simulink model "WorkingModel"  (R2023b)
settings: Solver=FixedStepDiscrete  StartTime=0.0  StopTime=param_sim_time  FixedStep=1/fs  MaxStep=1/fs  RelTol=1e-3
undefined symbols (not defined in the file): analyses, fdesignblkfcn, fs, gcbh, param_tot_samples
libraries: dspstat3 x13, SCGAnalysis_SignalGenerationLib x2
(part 2 of 20)

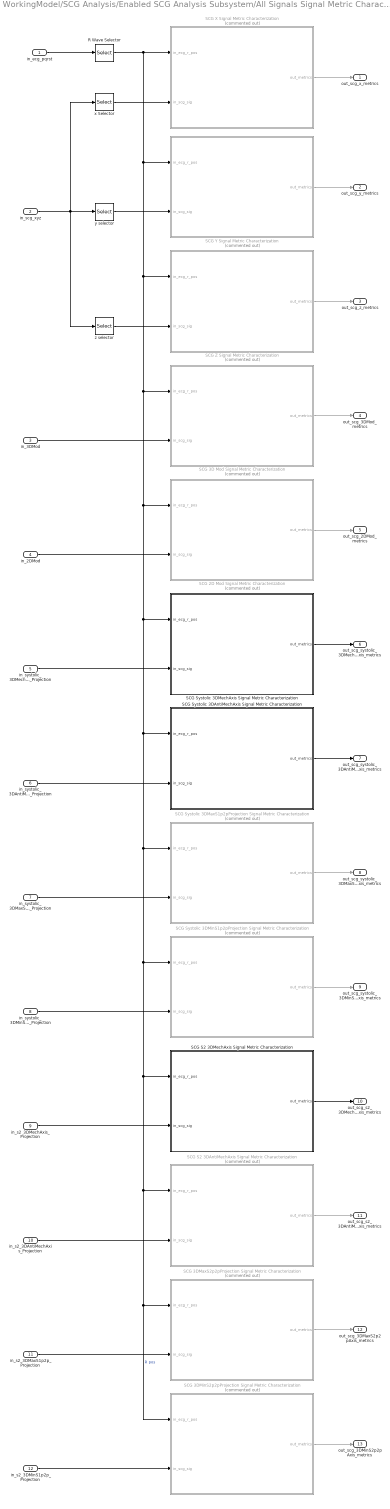
== system WorkingModel/SCG Analysis/Enabled SCG Analysis Subsystem/All Signals Signal Metric Characterization ==
  in_ecg_pqrst : Inport
  in_scg_xyz : Inport  Port=2
  in_3DMod : Inport  Port=3
  in_2DMod : Inport  Port=4
  in_systolic_3DMechAxis_Projection : Inport  Port=5
  in_systolic_3DAntiMechAxis_Projection : Inport  Port=6
  in_systolic_3DMaxS1p2p_Projection : Inport  Port=7
  in_systolic_3DMinS1p2p_Projection : Inport  Port=8
  in_s2_3DMechAxis_Projection : Inport  Port=9
  in_s2_3DAntiMechAxis_Projection : Inport  Port=10
  in_s2_3DMaxS1p2p_Projection : Inport  Port=11
  in_s2_3DMinS1p2p_Projection : Inport  Port=12
  R Wave Selector : Selector  NumberOfDimensions=2  InputPortWidth=3  IndexOptions=Select all,Index vector (dialog)  Indices=[1 3],3  OutputSizes=1,1
  SCG 2D Mod Signal Metric Characterization : Subsystem  Commented=on  mask{s1p2p_flag=on, s2p2p_flag=on, snr_flag=on, var_flag=on, morphvar_flag=on, nsd_flag=off}
      mask prompts: s1p2p_flag "S1 peak-to-peak Amplitude"; s2p2p_flag "S2 peak-to-peak Amplitude"; snr_flag "Signal-to-nose Ratio (can be further specified inside block)"; var_flag "Variance"; morphvar_flag "Cycle-to-cycle Morphological Variability"; nsd_flag "Normalized Spectral Distribution (can be further specified inside block)"
      mask DialogControl DescGroupVar Prompt: Signal Characterization
      mask DialogControl DescTextVar Prompt: SCG Signal Characterization block. Select which signal characterization metrics to evaluate:
      mask Display: image('C:\Users\Rafael\Dropbox\Post-Doc Research\Characterization.png'); % Use "Edit Image" on toolstrip to change.
  SCG 3D Mod Signal Metric Characterization : Subsystem  Commented=on  mask{s1p2p_flag=on, s2p2p_flag=on, snr_flag=on, var_flag=on, morphvar_flag=on, nsd_flag=off}
      mask prompts: s1p2p_flag "S1 peak-to-peak Amplitude"; s2p2p_flag "S2 peak-to-peak Amplitude"; snr_flag "Signal-to-nose Ratio (can be further specified inside block)"; var_flag "Variance"; morphvar_flag "Cycle-to-cycle Morphological Variability"; nsd_flag "Normalized Spectral Distribution (can be further specified inside block)"
      mask DialogControl DescGroupVar Prompt: Signal Characterization
      mask DialogControl DescTextVar Prompt: SCG Signal Characterization block. Select which signal characterization metrics to evaluate:
      mask Display: image('C:\Users\Rafael\Dropbox\Post-Doc Research\Characterization.png'); % Use "Edit Image" on toolstrip to change.
  SCG 3DMaxS2p2pProjection Signal Metric Characterization : Subsystem  Commented=on  mask{s1p2p_flag=on, s2p2p_flag=on, snr_flag=on, var_flag=on, morphvar_flag=on, nsd_flag=on}
      mask prompts: s1p2p_flag "S1 peak-to-peak Amplitude"; s2p2p_flag "S2 peak-to-peak Amplitude"; snr_flag "Signal-to-nose Ratio (can be further specified inside block)"; var_flag "Variance"; morphvar_flag "Cycle-to-cycle Morphological Variability"; nsd_flag "Normalized Spectral Distribution (can be further specified inside block)"
      mask DialogControl DescGroupVar Prompt: Signal Characterization
      mask DialogControl DescTextVar Prompt: SCG Signal Characterization block. Select which signal characterization metrics to evaluate:
      mask Display: image('C:\Users\Rafael\Dropbox\Post-Doc Research\Characterization.png'); % Use "Edit Image" on toolstrip to change.
  SCG 3DMinS2p2pProjection Signal Metric Characterization : Subsystem  Commented=on  mask{s1p2p_flag=on, s2p2p_flag=on, snr_flag=on, var_flag=on, morphvar_flag=on, nsd_flag=on}
      mask prompts: s1p2p_flag "S1 peak-to-peak Amplitude"; s2p2p_flag "S2 peak-to-peak Amplitude"; snr_flag "Signal-to-nose Ratio (can be further specified inside block)"; var_flag "Variance"; morphvar_flag "Cycle-to-cycle Morphological Variability"; nsd_flag "Normalized Spectral Distribution (can be further specified inside block)"
      mask DialogControl DescGroupVar Prompt: Signal Characterization
      mask DialogControl DescTextVar Prompt: SCG Signal Characterization block. Select which signal characterization metrics to evaluate:
      mask Display: image('C:\Users\Rafael\Dropbox\Post-Doc Research\Characterization.png'); % Use "Edit Image" on toolstrip to change.
  SCG S2 3DAntiMechAxis Signal Metric Characterization : Subsystem  Commented=on  mask{s1p2p_flag=on, s2p2p_flag=on, snr_flag=on, var_flag=on, morphvar_flag=on, nsd_flag=on}
      mask prompts: s1p2p_flag "S1 peak-to-peak Amplitude"; s2p2p_flag "S2 peak-to-peak Amplitude"; snr_flag "Signal-to-nose Ratio (can be further specified inside block)"; var_flag "Variance"; morphvar_flag "Cycle-to-cycle Morphological Variability"; nsd_flag "Normalized Spectral Distribution (can be further specified inside block)"
      mask DialogControl DescGroupVar Prompt: Signal Characterization
      mask DialogControl DescTextVar Prompt: SCG Signal Characterization block. Select which signal characterization metrics to evaluate:
      mask Display: image('C:\Users\Rafael\Dropbox\Post-Doc Research\Characterization.png'); % Use "Edit Image" on toolstrip to change.
  SCG S2 3DMechAxis Signal Metric Characterization : Subsystem  mask{s1p2p_flag=on, s2p2p_flag=on, snr_flag=on, var_flag=on, morphvar_flag=on, nsd_flag=on}
      mask prompts: s1p2p_flag "S1 peak-to-peak Amplitude"; s2p2p_flag "S2 peak-to-peak Amplitude"; snr_flag "Signal-to-nose Ratio (can be further specified inside block)"; var_flag "Variance"; morphvar_flag "Cycle-to-cycle Morphological Variability"; nsd_flag "Normalized Spectral Distribution (can be further specified inside block)"
      mask DialogControl DescGroupVar Prompt: Signal Characterization
      mask DialogControl DescTextVar Prompt: SCG Signal Characterization block. Select which signal characterization metrics to evaluate:
      mask Display: image('C:\Users\Rafael\Dropbox\Post-Doc Research\Characterization.png'); % Use "Edit Image" on toolstrip to change.
  SCG Systolic 3DAntiMechAxis Signal Metric Characterization : Subsystem  mask{s1p2p_flag=on, s2p2p_flag=on, snr_flag=on, var_flag=on, morphvar_flag=on, nsd_flag=on}
      mask prompts: s1p2p_flag "S1 peak-to-peak Amplitude"; s2p2p_flag "S2 peak-to-peak Amplitude"; snr_flag "Signal-to-nose Ratio (can be further specified inside block)"; var_flag "Variance"; morphvar_flag "Cycle-to-cycle Morphological Variability"; nsd_flag "Normalized Spectral Distribution (can be further specified inside block)"
      mask DialogControl DescGroupVar Prompt: Signal Characterization
      mask DialogControl DescTextVar Prompt: SCG Signal Characterization block. Select which signal characterization metrics to evaluate:
      mask Display: image('C:\Users\Rafael\Dropbox\Post-Doc Research\Characterization.png'); % Use "Edit Image" on toolstrip to change.
  SCG Systolic 3DMaxS1p2pProjection Signal Metric Characterization : Subsystem  Commented=on  mask{s1p2p_flag=on, s2p2p_flag=on, snr_flag=on, var_flag=on, morphvar_flag=on, nsd_flag=on}
      mask prompts: s1p2p_flag "S1 peak-to-peak Amplitude"; s2p2p_flag "S2 peak-to-peak Amplitude"; snr_flag "Signal-to-nose Ratio (can be further specified inside block)"; var_flag "Variance"; morphvar_flag "Cycle-to-cycle Morphological Variability"; nsd_flag "Normalized Spectral Distribution (can be further specified inside block)"
      mask DialogControl DescGroupVar Prompt: Signal Characterization
      mask DialogControl DescTextVar Prompt: SCG Signal Characterization block. Select which signal characterization metrics to evaluate:
      mask Display: image('C:\Users\Rafael\Dropbox\Post-Doc Research\Characterization.png'); % Use "Edit Image" on toolstrip to change.
  SCG Systolic 3DMechAxis Signal Metric Characterization : Subsystem  mask{s1p2p_flag=on, s2p2p_flag=on, snr_flag=on, var_flag=on, morphvar_flag=on, nsd_flag=on}
      mask prompts: s1p2p_flag "S1 peak-to-peak Amplitude"; s2p2p_flag "S2 peak-to-peak Amplitude"; snr_flag "Signal-to-nose Ratio (can be further specified inside block)"; var_flag "Variance"; morphvar_flag "Cycle-to-cycle Morphological Variability"; nsd_flag "Normalized Spectral Distribution (can be further specified inside block)"
      mask DialogControl DescGroupVar Prompt: Signal Characterization
      mask DialogControl DescTextVar Prompt: SCG Signal Characterization block. Select which signal characterization metrics to evaluate:
      mask Display: image('C:\Users\Rafael\Dropbox\Post-Doc Research\Characterization.png'); % Use "Edit Image" on toolstrip to change.
  SCG Systolic 3DMinS1p2pProjection Signal Metric Characterization : Subsystem  Commented=on  mask{s1p2p_flag=on, s2p2p_flag=on, snr_flag=on, var_flag=on, morphvar_flag=on, nsd_flag=on}
      mask prompts: s1p2p_flag "S1 peak-to-peak Amplitude"; s2p2p_flag "S2 peak-to-peak Amplitude"; snr_flag "Signal-to-nose Ratio (can be further specified inside block)"; var_flag "Variance"; morphvar_flag "Cycle-to-cycle Morphological Variability"; nsd_flag "Normalized Spectral Distribution (can be further specified inside block)"
      mask DialogControl DescGroupVar Prompt: Signal Characterization
      mask DialogControl DescTextVar Prompt: SCG Signal Characterization block. Select which signal characterization metrics to evaluate:
      mask Display: image('C:\Users\Rafael\Dropbox\Post-Doc Research\Characterization.png'); % Use "Edit Image" on toolstrip to change.
  SCG X Signal Metric Characterization : Subsystem  Commented=on  mask{s1p2p_flag=on, s2p2p_flag=on, snr_flag=on, var_flag=on, morphvar_flag=on, nsd_flag=on}
      mask prompts: s1p2p_flag "S1 peak-to-peak Amplitude"; s2p2p_flag "S2 peak-to-peak Amplitude"; snr_flag "Signal-to-nose Ratio (can be further specified inside block)"; var_flag "Variance"; morphvar_flag "Cycle-to-cycle Morphological Variability"; nsd_flag "Normalized Spectral Distribution (can be further specified inside block)"
      mask DialogControl DescGroupVar Prompt: Signal Characterization
      mask DialogControl DescTextVar Prompt: SCG Signal Characterization block. Select which signal characterization metrics to evaluate:
      mask Display: image('C:\Users\Rafael\Dropbox\Post-Doc Research\Characterization.png'); % Use "Edit Image" on toolstrip to change.
  SCG Y Signal Metric Characterization : Subsystem  Commented=on  mask{s1p2p_flag=on, s2p2p_flag=on, snr_flag=on, var_flag=on, morphvar_flag=on, nsd_flag=on}
      mask prompts: s1p2p_flag "S1 peak-to-peak Amplitude"; s2p2p_flag "S2 peak-to-peak Amplitude"; snr_flag "Signal-to-nose Ratio (can be further specified inside block)"; var_flag "Variance"; morphvar_flag "Cycle-to-cycle Morphological Variability"; nsd_flag "Normalized Spectral Distribution (can be further specified inside block)"
      mask DialogControl DescGroupVar Prompt: Signal Characterization
      mask DialogControl DescTextVar Prompt: SCG Signal Characterization block. Select which signal characterization metrics to evaluate:
      mask Display: image('C:\Users\Rafael\Dropbox\Post-Doc Research\Characterization.png'); % Use "Edit Image" on toolstrip to change.
  SCG Z Signal Metric Characterization : Subsystem  Commented=on  mask{s1p2p_flag=on, s2p2p_flag=on, snr_flag=on, var_flag=on, morphvar_flag=on, nsd_flag=on}
      mask prompts: s1p2p_flag "S1 peak-to-peak Amplitude"; s2p2p_flag "S2 peak-to-peak Amplitude"; snr_flag "Signal-to-nose Ratio (can be further specified inside block)"; var_flag "Variance"; morphvar_flag "Cycle-to-cycle Morphological Variability"; nsd_flag "Normalized Spectral Distribution (can be further specified inside block)"
      mask DialogControl DescGroupVar Prompt: Signal Characterization
      mask DialogControl DescTextVar Prompt: SCG Signal Characterization block. Select which signal characterization metrics to evaluate:
      mask Display: image('C:\Users\Rafael\Dropbox\Post-Doc Research\Characterization.png'); % Use "Edit Image" on toolstrip to change.
  x Selector : Selector  NumberOfDimensions=2  InputPortWidth=3  IndexOptions=Select all,Index vector (dialog)  Indices=[1 3],[1]  OutputSizes=1,1
  y selector : Selector  NumberOfDimensions=2  InputPortWidth=3  IndexOptions=Select all,Index vector (dialog)  Indices=[1 3],[2]  OutputSizes=1,1
  z selector : Selector  NumberOfDimensions=2  InputPortWidth=3  IndexOptions=Select all,Index vector (dialog)  Indices=[1 3],[3]  OutputSizes=1,1
  out_scg_x_metrics : Outport
  out_scg_y_metrics : Outport  Port=2
  out_scg_z_metrics : Outport  Port=3
  out_scg_3DMod_metrics : Outport  Port=4
  out_scg_2DMod_metrics : Outport  Port=5
  out_scg_systolic_3DMechAxis_metrics : Outport  Port=6
  out_scg_systolic_3DAntiMechAxis_metrics : Outport  Port=7
  out_scg_systolic_3DMaxS1p2pAxis_metrics : Outport  Port=8
  out_scg_systolic_3DMinS1p2pAxis_metrics : Outport  Port=9
  out_scg_s2_3DMechAxis_metrics : Outport  Port=10
  out_scg_s2_3DAntiMechAxis_metrics : Outport  Port=11
  out_scg_3DMaxS2p2pAxis_metrics : Outport  Port=12
  out_scg_3DMinS2p2pAxis_metrics : Outport  Port=13
  wires:
  in_scg_xyz/1 -> y selector/1, z selector/1, x Selector/1
  x Selector/1 -> SCG X Signal Metric Characterization/2(in_scg_sig)
  in_ecg_pqrst/1 -> R Wave Selector/1
  R Wave Selector/1 -> SCG Systolic 3DAntiMechAxis Signal Metric Characterization/1(in_ecg_r_pos), SCG Systolic 3DMaxS1p2pProjection Signal Metric Characterization/1(in_ecg_r_pos), SCG 3DMinS2p2pProjection Signal Metric Characterization/1(in_ecg_r_pos), SCG 3DMaxS2p2pProjection Signal Metric Characterization/1(in_ecg_r_pos), SCG S2 3DAntiMechAxis Signal Metric Characterization/1(in_ecg_r_pos), SCG S2 3DMechAxis Signal Metric Characterization/1(in_ecg_r_pos), SCG Systolic 3DMinS1p2pProjection Signal Metric Characterization/1(in_ecg_r_pos), SCG Systolic 3DMechAxis Signal Metric Characterization/1(in_ecg_r_pos), SCG 2D Mod Signal Metric Characterization/1(in_ecg_r_pos), SCG 3D Mod Signal Metric Characterization/1(in_ecg_r_pos), SCG Z Signal Metric Characterization/1(in_ecg_r_pos), SCG Y Signal Metric Characterization/1(in_ecg_r_pos), SCG X Signal Metric Characterization/1(in_ecg_r_pos)  "R pos"
  y selector/1 -> SCG Y Signal Metric Characterization/2(in_scg_sig)
  z selector/1 -> SCG Z Signal Metric Characterization/2(in_scg_sig)
  SCG X Signal Metric Characterization/1(out_metrics) -> out_scg_x_metrics/1
  SCG Y Signal Metric Characterization/1(out_metrics) -> out_scg_y_metrics/1
  SCG Z Signal Metric Characterization/1(out_metrics) -> out_scg_z_metrics/1
  in_3DMod/1 -> SCG 3D Mod Signal Metric Characterization/2(in_scg_sig)
  SCG 3D Mod Signal Metric Characterization/1(out_metrics) -> out_scg_3DMod_metrics/1
  in_2DMod/1 -> SCG 2D Mod Signal Metric Characterization/2(in_scg_sig)
  SCG 2D Mod Signal Metric Characterization/1(out_metrics) -> out_scg_2DMod_metrics/1
  in_systolic_3DMechAxis_Projection/1 -> SCG Systolic 3DMechAxis Signal Metric Characterization/2(in_scg_sig)
  SCG Systolic 3DMechAxis Signal Metric Characterization/1(out_metrics) -> out_scg_systolic_3DMechAxis_metrics/1
  in_systolic_3DAntiMechAxis_Projection/1 -> SCG Systolic 3DAntiMechAxis Signal Metric Characterization/2(in_scg_sig)
  SCG Systolic 3DAntiMechAxis Signal Metric Characterization/1(out_metrics) -> out_scg_systolic_3DAntiMechAxis_metrics/1
  in_systolic_3DMaxS1p2p_Projection/1 -> SCG Systolic 3DMaxS1p2pProjection Signal Metric Characterization/2(in_scg_sig)
  SCG Systolic 3DMaxS1p2pProjection Signal Metric Characterization/1(out_metrics) -> out_scg_systolic_3DMaxS1p2pAxis_metrics/1
  in_systolic_3DMinS1p2p_Projection/1 -> SCG Systolic 3DMinS1p2pProjection Signal Metric Characterization/2(in_scg_sig)
  SCG Systolic 3DMinS1p2pProjection Signal Metric Characterization/1(out_metrics) -> out_scg_systolic_3DMinS1p2pAxis_metrics/1
  SCG S2 3DMechAxis Signal Metric Characterization/1(out_metrics) -> out_scg_s2_3DMechAxis_metrics/1
  SCG 3DMinS2p2pProjection Signal Metric Characterization/1(out_metrics) -> out_scg_3DMinS2p2pAxis_metrics/1
  SCG S2 3DAntiMechAxis Signal Metric Characterization/1(out_metrics) -> out_scg_s2_3DAntiMechAxis_metrics/1
  SCG 3DMaxS2p2pProjection Signal Metric Characterization/1(out_metrics) -> out_scg_3DMaxS2p2pAxis_metrics/1
  in_s2_3DMinS1p2p_Projection/1 -> SCG 3DMinS2p2pProjection Signal Metric Characterization/2(in_scg_sig)
  in_s2_3DMaxS1p2p_Projection/1 -> SCG 3DMaxS2p2pProjection Signal Metric Characterization/2(in_scg_sig)
  in_s2_3DAntiMechAxis_Projection/1 -> SCG S2 3DAntiMechAxis Signal Metric Characterization/2(in_scg_sig)
  in_s2_3DMechAxis_Projection/1 -> SCG S2 3DMechAxis Signal Metric Characterization/2(in_scg_sig)

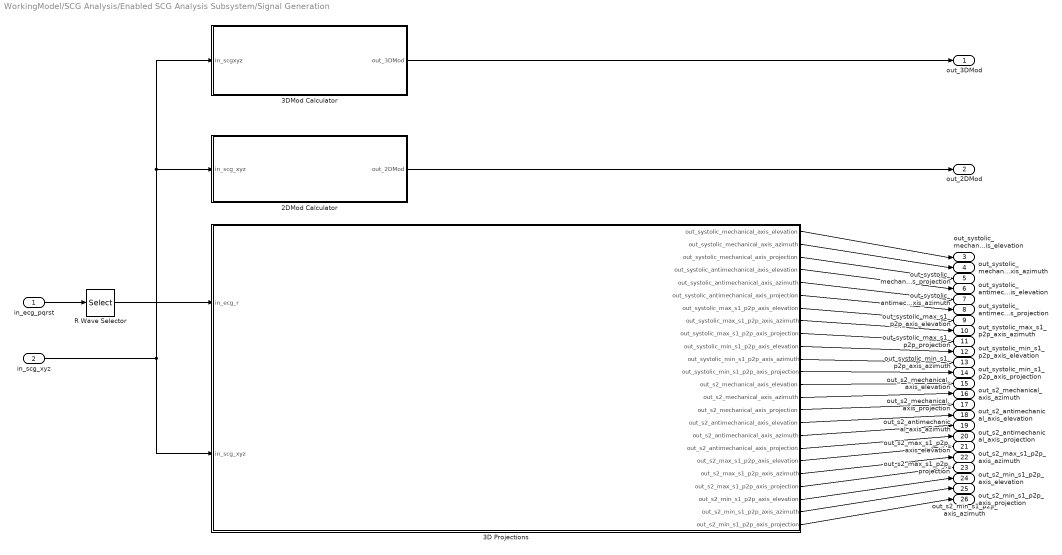
== system WorkingModel/SCG Analysis/Enabled SCG Analysis Subsystem/Signal Generation ==
  in_ecg_pqrst : Inport
  in_scg_xyz : Inport  Port=2
  2DMod Calculator : Subsystem  mask{xyz2Dcombo=xz (transverse plane)}
      mask prompts: xyz2Dcombo "2D component combination:"
      mask init:
      | if xyz2Dcombo == 1
      |     param_2Dxyzcombo = 'xy';
      | elseif xyz2Dcombo == 2
      |     param_2Dxyzcombo = 'yz';
      | elseif xyz2Dcombo == 3
      |     param_2Dxyzcombo = 'xz';
      | end
      | 
      | assignin('base','param_2Dxyzcombo', param_2Dxyzcombo)
      mask TypeOptions xyz2Dcombo: xy (coronal plane) | yz (sagittal plane) | xz (transverse plane)
      mask DialogControl DescGroupVar Prompt: 2D Modulus Calculator
      mask DialogControl DescTextVar Prompt: Subsystem to calculate a 2D modulus signal from a user-specified combination of any two of the SCG x, y, or z components.
  3D Projections : Subsystem
      mask Display: image('C:\Users\Rafael\Dropbox\Post-Doc Research\Coordinate Frames with Signals.png'); % Use "Edit Image" on toolstrip to change.
  3DMod Calculator : Subsystem
  R Wave Selector : Selector  NumberOfDimensions=2  InputPortWidth=3  IndexOptions=Select all,Index vector (dialog)  Indices=[1 3],3  OutputSizes=1,1
  out_3DMod : Outport
  out_2DMod : Outport  Port=2
  out_systolic_mechanical_axis_elevation : Outport  Port=3
  out_systolic_mechanical_axis_azimuth : Outport  Port=4
  out_systolic_mechanical_axis_projection : Outport  Port=5
  out_systolic_antimechanical_axis_elevation : Outport  Port=6
  out_systolic_antimechanical_axis_azimuth : Outport  Port=7
  out_systolic_antimechanical_axis_projection : Outport  Port=8
  out_systolic_max_s1_p2p_axis_elevation : Outport  Port=9
  out_systolic_max_s1_p2p_axis_azimuth : Outport  Port=10
  out_systolic_max_s1_p2p_projection : Outport  Port=11
  out_systolic_min_s1_p2p_axis_elevation : Outport  Port=12
  out_systolic_min_s1_p2p_axis_azimuth : Outport  Port=13
  out_systolic_min_s1_p2p_axis_projection : Outport  Port=14
  out_s2_mechanical_axis_elevation : Outport  Port=15
  out_s2_mechanical_axis_azimuth : Outport  Port=16
  out_s2_mechanical_axis_projection : Outport  Port=17
  out_s2_antimechanical_axis_elevation : Outport  Port=18
  out_s2_antimechanical_axis_azimuth : Outport  Port=19
  out_s2_antimechanical_axis_projection : Outport  Port=20
  out_s2_max_s1_p2p_axis_elevation : Outport  Port=21
  out_s2_max_s1_p2p_axis_azimuth : Outport  Port=22
  out_s2_max_s1_p2p_projection : Outport  Port=23
  out_s2_min_s1_p2p_axis_elevation : Outport  Port=24
  out_s2_min_s1_p2p_axis_azimuth : Outport  Port=25
  out_s2_min_s1_p2p_axis_projection : Outport  Port=26
  wires:
  3DMod Calculator/1(out_3DMod) -> out_3DMod/1
  2DMod Calculator/1(out_2DMod) -> out_2DMod/1
  R Wave Selector/1 -> 3D Projections/1(in_ecg_r)
  in_ecg_pqrst/1 -> R Wave Selector/1
  in_scg_xyz/1 -> 2DMod Calculator/1(in_scg_xyz), 3DMod Calculator/1(in_scgxyz), 3D Projections/2(in_scg_xyz)
  3D Projections/4(out_systolic_antimechanical_axis_elevation) -> out_systolic_antimechanical_axis_elevation/1
  3D Projections/2(out_systolic_mechanical_axis_azimuth) -> out_systolic_mechanical_axis_azimuth/1
  3D Projections/10(out_systolic_min_s1_p2p_axis_elevation) -> out_systolic_min_s1_p2p_axis_elevation/1
  3D Projections/5(out_systolic_antimechanical_axis_azimuth) -> out_systolic_antimechanical_axis_azimuth/1
  3D Projections/8(out_systolic_max_s1_p2p_axis_azimuth) -> out_systolic_max_s1_p2p_axis_azimuth/1
  3D Projections/6(out_systolic_antimechanical_axis_projection) -> out_systolic_antimechanical_axis_projection/1
  3D Projections/7(out_systolic_max_s1_p2p_axis_elevation) -> out_systolic_max_s1_p2p_axis_elevation/1
  3D Projections/11(out_systolic_min_s1_p2p_axis_azimuth) -> out_systolic_min_s1_p2p_axis_azimuth/1
  3D Projections/12(out_systolic_min_s1_p2p_axis_projection) -> out_systolic_min_s1_p2p_axis_projection/1
  3D Projections/9(out_systolic_max_s1_p2p_axis_projection) -> out_systolic_max_s1_p2p_projection/1
  3D Projections/1(out_systolic_mechanical_axis_elevation) -> out_systolic_mechanical_axis_elevation/1
  3D Projections/3(out_systolic_mechanical_axis_projection) -> out_systolic_mechanical_axis_projection/1
  3D Projections/13(out_s2_mechanical_axis_elevation) -> out_s2_mechanical_axis_elevation/1
  3D Projections/14(out_s2_mechanical_axis_azimuth) -> out_s2_mechanical_axis_azimuth/1
  3D Projections/15(out_s2_mechanical_axis_projection) -> out_s2_mechanical_axis_projection/1
  3D Projections/16(out_s2_antimechanical_axis_elevation) -> out_s2_antimechanical_axis_elevation/1
  3D Projections/17(out_s2_antimechanical_axis_azimuth) -> out_s2_antimechanical_axis_azimuth/1
  3D Projections/18(out_s2_antimechanical_axis_projection) -> out_s2_antimechanical_axis_projection/1
  3D Projections/19(out_s2_max_s1_p2p_axis_elevation) -> out_s2_max_s1_p2p_axis_elevation/1
  3D Projections/20(out_s2_max_s1_p2p_axis_azimuth) -> out_s2_max_s1_p2p_axis_azimuth/1
  3D Projections/21(out_s2_max_s1_p2p_axis_projection) -> out_s2_max_s1_p2p_projection/1
  3D Projections/22(out_s2_min_s1_p2p_axis_elevation) -> out_s2_min_s1_p2p_axis_elevation/1
  3D Projections/23(out_s2_min_s1_p2p_axis_azimuth) -> out_s2_min_s1_p2p_axis_azimuth/1
  3D Projections/24(out_s2_min_s1_p2p_axis_projection) -> out_s2_min_s1_p2p_axis_projection/1

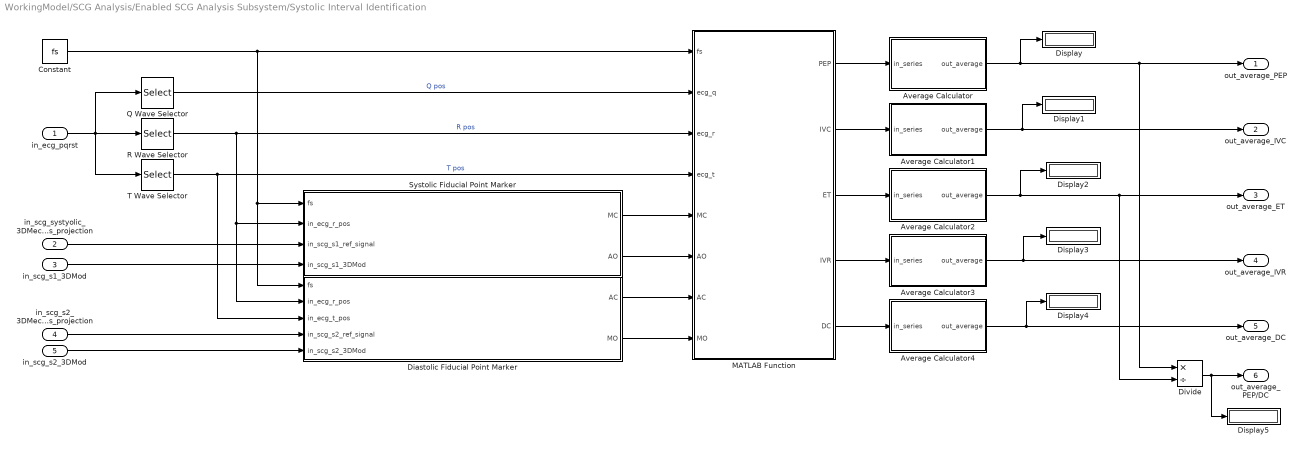
== system WorkingModel/SCG Analysis/Enabled SCG Analysis Subsystem/Systolic Interval Identification ==
  in_ecg_pqrst : Inport
  in_scg_systyolic_3DMechAxis_projection : Inport  Port=2
  in_scg_s1_3DMod : Inport  Port=3
  in_scg_s2_3DMechAxis_projection : Inport  Port=4
  in_scg_s2_3DMod : Inport  Port=5
  Average Calculator : Subsystem  mask{average_type=Median}
      mask TypeOptions average_type: Mean | Median | Mode
      mask DialogControl DescGroupVar Prompt: Average Calculator
      mask DialogControl DescTextVar Prompt: Select the type of average you wish to calculate:
  Average Calculator1 : Subsystem  mask{average_type=Median}
      mask TypeOptions average_type: Mean | Median | Mode
      mask DialogControl DescGroupVar Prompt: Average Calculator
      mask DialogControl DescTextVar Prompt: Select the type of average you wish to calculate:
  Average Calculator2 : Subsystem  mask{average_type=Median}
      mask TypeOptions average_type: Mean | Median | Mode
      mask DialogControl DescGroupVar Prompt: Average Calculator
      mask DialogControl DescTextVar Prompt: Select the type of average you wish to calculate:
  Average Calculator3 : Subsystem  mask{average_type=Median}
      mask TypeOptions average_type: Mean | Median | Mode
      mask DialogControl DescGroupVar Prompt: Average Calculator
      mask DialogControl DescTextVar Prompt: Select the type of average you wish to calculate:
  Average Calculator4 : Subsystem  mask{average_type=Median}
      mask TypeOptions average_type: Mean | Median | Mode
      mask DialogControl DescGroupVar Prompt: Average Calculator
      mask DialogControl DescTextVar Prompt: Select the type of average you wish to calculate:
  Constant : Constant  Value=fs
  Diastolic Fiducial Point Marker : Subsystem
  Display{,1..5} (6 alike) : Display
  Divide : Product  Inputs=*/
  MATLAB Function : MATLAB Function  TreatAsAtomicUnit=on
  Q Wave Selector : Selector  NumberOfDimensions=2  InputPortWidth=3  IndexOptions=Select all,Index vector (dialog)  Indices=[1 3],2  OutputSizes=1,1
  R Wave Selector : Selector  NumberOfDimensions=2  InputPortWidth=3  IndexOptions=Select all,Index vector (dialog)  Indices=[1 3],3  OutputSizes=1,1
  Systolic Fiducial Point Marker : Subsystem
  T Wave Selector : Selector  NumberOfDimensions=2  InputPortWidth=3  IndexOptions=Select all,Index vector (dialog)  Indices=[1 3],5  OutputSizes=1,1
  out_average_PEP : Outport
  out_average_IVC : Outport  Port=2
  out_average_ET : Outport  Port=3
  out_average_IVR : Outport  Port=4
  out_average_DC : Outport  Port=5
  out_average_PEP/DC : Outport  Port=6
  wires:
  in_ecg_pqrst/1 -> Q Wave Selector/1, T Wave Selector/1, R Wave Selector/1
  Constant/1 -> MATLAB Function/1(fs), Diastolic Fiducial Point Marker/1(fs), Systolic Fiducial Point Marker/1(fs)
  R Wave Selector/1 -> MATLAB Function/3(ecg_r), Diastolic Fiducial Point Marker/2(in_ecg_r_pos), Systolic Fiducial Point Marker/2(in_ecg_r_pos)  "R pos"
  in_scg_systyolic_3DMechAxis_projection/1 -> Systolic Fiducial Point Marker/3(in_scg_s1_ref_signal)
  in_scg_s1_3DMod/1 -> Systolic Fiducial Point Marker/4(in_scg_s1_3DMod)
  in_scg_s2_3DMechAxis_projection/1 -> Diastolic Fiducial Point Marker/4(in_scg_s2_ref_signal)
  in_scg_s2_3DMod/1 -> Diastolic Fiducial Point Marker/5(in_scg_s2_3DMod)
  T Wave Selector/1 -> MATLAB Function/4(ecg_t), Diastolic Fiducial Point Marker/3(in_ecg_t_pos)  "T pos"
  Q Wave Selector/1 -> MATLAB Function/2(ecg_q)  "Q pos"
  Systolic Fiducial Point Marker/1(MC) -> MATLAB Function/5(MC)
  Systolic Fiducial Point Marker/2(AO) -> MATLAB Function/6(AO)
  Diastolic Fiducial Point Marker/1(AC) -> MATLAB Function/7(AC)
  Diastolic Fiducial Point Marker/2(MO) -> MATLAB Function/8(MO)
  MATLAB Function/1(PEP) -> Average Calculator/1(in_series)
  MATLAB Function/2(IVC) -> Average Calculator1/1(in_series)
  MATLAB Function/3(ET) -> Average Calculator2/1(in_series)
  MATLAB Function/4(IVR) -> Average Calculator3/1(in_series)
  MATLAB Function/5(DC) -> Average Calculator4/1(in_series)
  Average Calculator/1(out_average) -> Divide/1, out_average_PEP/1, Display/1
  Average Calculator1/1(out_average) -> Display1/1, out_average_IVC/1
  Average Calculator2/1(out_average) -> Display2/1, Divide/2, out_average_ET/1
  Average Calculator3/1(out_average) -> Display3/1, out_average_IVR/1
  Average Calculator4/1(out_average) -> Display4/1, out_average_DC/1
  Divide/1 -> Display5/1, out_average_PEP/DC/1

== system WorkingModel/SCG Preprocessing/Enabled SCG Preprocessing Subsystem/Filtfiltering ==
  " input SCG" : Inport
  Bandpass Filter 1 : Subsystem  DialogController=fdesignblkfcn  InitFcn=fdesignblkfcn(gcbh, {'InitFcn'});  mask(Bandpass Filter){}
      mask help: Design a bandpass filter
      settings: CopyFcn=fdesignblkfcn(gcbh, {'CopyFcn'});
      mask Help: helpview(mapfilelocation('dsp'), 'dspbandpassfilter');
      mask Display: disp('Bandpass');
  Bandpass Filter 2 : Subsystem  DialogController=fdesignblkfcn  InitFcn=fdesignblkfcn(gcbh, {'InitFcn'});  mask(Bandpass Filter){}
      mask help: Design a bandpass filter
      settings: CopyFcn=fdesignblkfcn(gcbh, {'CopyFcn'});
      mask Help: helpview(mapfilelocation('dsp'), 'dspbandpassfilter');
      mask Display: disp('Bandpass');
  Flip : DSPFlip
  Flip1 : DSPFlip
  filtfiltered SCG : Outport  VectorParamsAs1DForOutWhenUnconnected=off
  wires:
  Bandpass Filter 2/1(Out) -> Flip1/1
  Bandpass Filter 1/1(Out) -> Flip/1
  Flip1/1 -> filtfiltered SCG/1
  " input SCG"/1 -> Bandpass Filter 1/1(In)
  Flip/1 -> Bandpass Filter 2/1(In)

== system WorkingModel/SCG Preprocessing/Enabled SCG Preprocessing Subsystem/To Workspace: Processed SCGxyz ==
  In1 : Inport
  To Workspace SCG Enabled Subsystem : Subsystem  TreatAsAtomicUnit=on
  wires:
  In1/1 -> To Workspace SCG Enabled Subsystem/Enable, To Workspace SCG Enabled Subsystem/1(In1)

== system WorkingModel/ECG Analysis/Enabled ECG Analysis Subsystem/Assign To Workspace: Num Cycles/Enabled To Workspace ECG Num Cycles ==
  note: Make sure the funtion expects input dimensions of appropriate size.
  note: The subsystem is only enabled when it receives a (non-zero) signal
  Enable : EnablePort  ShowOutputPort=on
  Slk Wrapped Assigned To Workspace : MATLAB Function  TreatAsAtomicUnit=on
  wires:
  Enable/1 -> Slk Wrapped Assigned To Workspace/1(assigned_var)

== system WorkingModel/ECG Analysis/Enabled ECG Analysis Subsystem/Assign To Workspace: idxs PQRST/Enabled To Workspace idxs PQRST ==
  note: Make sure the funtion expects input dimensions of appropriate size.
  note: The subsystem is only enabled when it receives a (non-zero) signal
  in_idxs_pqrst : Inport
  Enable : EnablePort
  Slk Wrapped Assigned to Workspace : MATLAB Function  TreatAsAtomicUnit=on
  wires:
  in_idxs_pqrst/1 -> Slk Wrapped Assigned to Workspace/1(idxs_pqrst)
